simulink model "SpheroControl_CVT"  (R2014b)
settings: Solver=ode3  StartTime=0.0  StopTime=30  FixedStep=.2  RelTol=1e-3
InitFcn:
  | %sphName = uint8('Sphero-PGP');
  | 
  | move(char(sphName), 0, 0)
  | 
  | restartspeed = 65;
  | stopspeed = 1;
  | stopRadius = 50;
  | Kp = 0.2;
  |     Ki = 0;
  |     Kd = 0;
StopFcn:
  | %detectSpheroCVT( 10, 1);
  | 
  | move(sphName, 0, 0)
  | move(sphName, 0, 0, 0)
undefined symbols (not defined in the file or in its folder): IsPositionTracked, IsSkeletonTracked, JointDepthIndices, JointImageIndices, JointTrackingState, JointWorldCoordinates, none, PositionDepthIndices, PositionImageIndices, PositionWorldCoordinates, SegmentationData, SkeletonTrackingID, videoinput
libraries: visiontextngfix x1, imaqlib x1, aerolibanimutils x1, visionsinks x1
settings Model: Creator=dsethi  LastModifiedBy=dsethi
settings SolverCC: AlgebraicLoopSolver=LineSearch
settings DataIOCC: SignalLoggingSaveFormat=ModelDataLogs
settings DebuggingCC: MultiTaskDSMMsg=warning  MultiTaskCondExecSysMsg=none
settings RTWCC: IncludeERTFirstTime=on

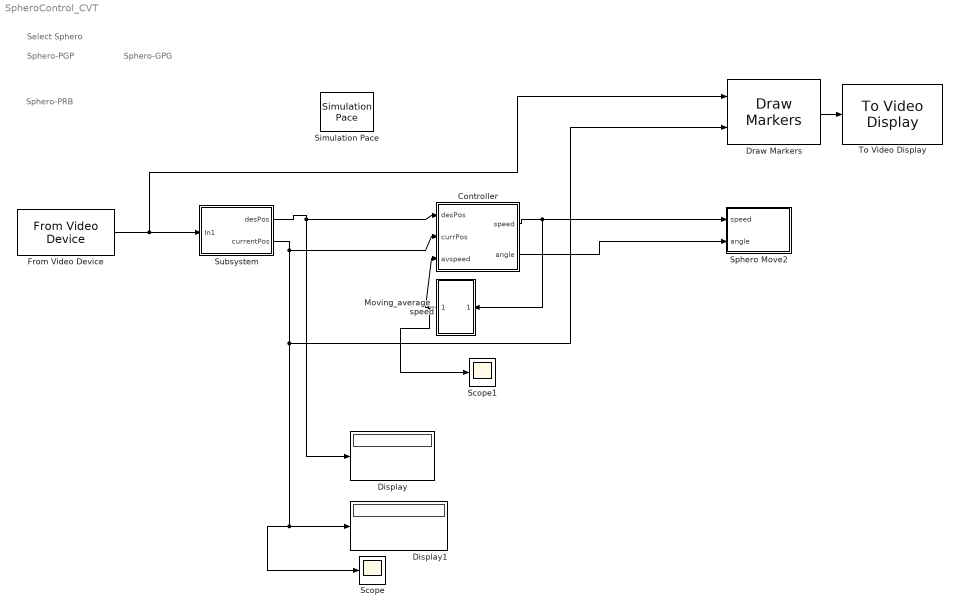
== system SpheroControl_CVT ==
  note: Select Sphero
  note: Sphero-PGP
  note: Sphero-GPG
  note: Sphero-PRB
  Controller : Stateflow chart  TreatAsAtomicUnit=on
  Display : Display
  Display1 : Display
  Draw Markers : visiontextngfix/Draw Markers  shape=X-mark  size=3  fill=off  fillClrSource=Specify via dialog  display=User-specified value  intensity=200  color=[255 0 0]  opacity=0.6  viewport=Entire image  antialiasing=off  inType=Obsolete  imagePorts=One multidimensional signal  prodOutputMode=Binary point scaling  prodOutputWordLength=32  prodOutputFracLength=14  memoryMode=Specify word length  memoryWordLength=16  memoryFracLength=15  roundingMode=Floor  overflowMode=off
  From Video Device : imaqlib/From Video Device  DeviceMenu=winvideo 1 (Microsoft LifeCam Cinema)  Device=winvideo 1 (Microsoft LifeCam Cinema)  ObjConstructor=videoinput('winvideo', 1)  VideoFormatMenu=MJPG_640x480  VideoFormat=MJPG_640x480  VideoSource=input1  ROIPosition=[0 0 480 640]  EnableHWTrigger=off  TriggerConfiguration=none/none  SampleTime=0.2  OutputPortsMode=One multidimensional signal  DataType=single  CanDoHWTrigger=no  ReturnedColorSpace=rgb  BlockHandle=1921.0006  ROIWidth=640  ROIHeight=480  ROIColumn=0  ROIRow=0  EngXMLPath=D:\jobarchive\R2014bd\2014_07_22_h06m43s29_job123_pass\matlab\toolbox\imaq\imaq\private  DevXMLPath=D:\jobarchive\R2014bd\2014_07_22_h06m43s29_job123_pass\matlab\toolbox\imaq\supportpackages\genericvideo\adaptor\win64  EngLibPath=D:\jobarchive\R2014bd\2014_07_22_h06m43s29_job123_pass\matlab\toolbox\imaq\imaqblks\imaqmex\win64  ColorSpace=rgb  BayerSensorAlignment=grbg  AllMetadata=IsPositionTracked;IsSkeletonTracked;JointDepthIndices;JointImageIndices;JointTrackingState;JointWorldCoordinates;PositionDepthIndices;PositionImageIndices;PositionWorldCoordinates;SegmentationData;SkeletonTrackingID
  Moving_average_speed : Subsystem
  Scope : Scope
      settings: SaveName=SpheroPos
  Scope1 : Scope
      settings: SaveName=movingAvg
  Simulation Pace : aerolibanimutils/Simulation Pace  SimulationPace=1  SleepMode=MATLAB Thread  OutputPaceError=off  SampleTime=-1
      settings: AttributesFormatString=%<SimulationPace> sec/sec
  Sphero Move2 : MATLAB Function  TreatAsAtomicUnit=on
  Subsystem : Subsystem  mask{cameraNum=Logitech, desPos=[200, 150]}
      mask prompts: cameraNum "Camera"; desPos "Desired position (x, y coordinates)"
      mask TypeOptions cameraNum: Logitech | Microsoft
  To Video Display : visionsinks/To Video Display  inputType=Obsolete  imagePorts=One multidimensional signal  OutputDevice=On-screen video monitor  fullScreen=off  videoWindowX=-7  videoWindowY=10  saveWindowSize=off  videoWindowWidth=640  videoWindowHeight=480  dataOrg=Column-major  openAtMdlStart=on  isWindowOpen=off  inputColorFormat=RGB
  wires:
  Subsystem/1(desPos) -> Display/1, Controller/1(desPos)
  Subsystem/2(currentPos) -> Controller/2(currPos), Scope/1, Display1/1, Draw Markers/2
  From Video Device/1 -> Draw Markers/1, Subsystem/1(In1)
  Draw Markers/1 -> To Video Display/1
  Controller/1(speed) -> Moving_average_speed/1(In1), Sphero Move2/1(speed)
  Controller/2(angle) -> Sphero Move2/2(angle)
  Moving_average_speed/1(Out1) -> Scope1/1, Controller/3(avspeed)

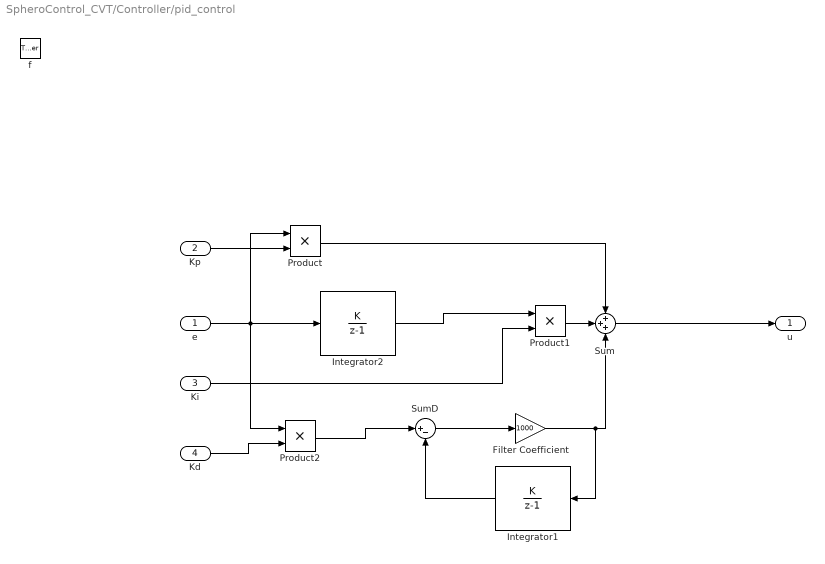
== system SpheroControl_CVT/Controller/pid_control ==
  e : Inport  OutDataTypeStr=double  PortDimensions=1
  Kp : Inport  Port=2  OutDataTypeStr=double  PortDimensions=1
  Ki : Inport  Port=3  OutDataTypeStr=double  PortDimensions=1
  Kd : Inport  Port=4  OutDataTypeStr=double  PortDimensions=1
  f : TriggerPort  TriggerType=function-call
      settings: CopyFcn=Stateflow.SLINSF.SimulinkMan.removeBlockPreDeleteFcn  PreDeleteFcn=Stateflow.SLINSF.SimulinkMan.unsafePredeleteFcn
  Filter Coefficient : Gain  Gain=1000
  Integrator1 : DiscreteIntegrator  IntegratorMethod=Accumulation: Forward Euler  InitialConditionSetting=State (most efficient)  SampleTime=-1
  Integrator2 : DiscreteIntegrator  IntegratorMethod=Accumulation: Forward Euler  InitialConditionSetting=State (most efficient)  SampleTime=-1
  Product : Product
  Product1 : Product
  Product2 : Product
  Sum : Sum  Inputs=+++
  SumD : Sum  DisableCoverage=on  Inputs=|+-
  u : Outport
  wires:
  Sum/1 -> u/1
  Product1/1 -> Sum/2
  Integrator1/1 -> SumD/2
  Filter Coefficient/1 -> Integrator1/1, Sum/3
  SumD/1 -> Filter Coefficient/1
  Product2/1 -> SumD/1
  Product/1 -> Sum/1
  e/1 -> Integrator2/1, Product2/1, Product/1
  Kp/1 -> Product/2
  Integrator2/1 -> Product1/1
  Ki/1 -> Product1/2
  Kd/1 -> Product2/2

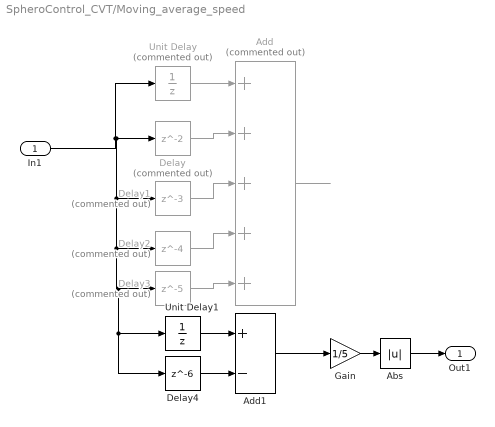
== system SpheroControl_CVT/Moving_average_speed ==
  In1 : Inport
  Abs : Abs
  Add : Sum  Commented=on  Inputs=+++++
  Add1 : Sum  Inputs=+-
  Delay : Delay  Commented=on
  Delay1 : Delay  Commented=on  DelayLength=3
  Delay2 : Delay  Commented=on  DelayLength=4
  Delay3 : Delay  Commented=on  DelayLength=5
  Delay4 : Delay  DelayLength=6
  Gain : Gain  Gain=1/5
  Unit Delay : UnitDelay  Commented=on  SampleTime=-1
  Unit Delay1 : UnitDelay  SampleTime=-1
  Out1 : Outport
  wires:
  Delay/1 -> Add/2
  In1/1 -> Unit Delay/1, Unit Delay1/1, Delay4/1, Delay3/1, Delay2/1, Delay1/1, Delay/1
  Unit Delay/1 -> Add/1
  Delay1/1 -> Add/3
  Delay2/1 -> Add/4
  Delay3/1 -> Add/5
  Add/1 -> ?
  Gain/1 -> Abs/1
  Delay4/1 -> Add1/2
  Add1/1 -> Gain/1
  Unit Delay1/1 -> Add1/1
  Abs/1 -> Out1/1

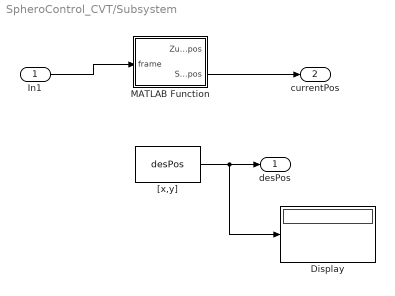
== system SpheroControl_CVT/Subsystem ==
  In1 : Inport
  Display : Display
  MATLAB Function : MATLAB Function  TreatAsAtomicUnit=on
  "[x,y]" : Constant  Value=desPos
  desPos : Outport
  currentPos : Outport  Port=2
  wires:
  "[x,y]"/1 -> Display/1, desPos/1
  In1/1 -> MATLAB Function/1(frame)
  MATLAB Function/2(Spheropos) -> currentPos/1

== matlab function SpheroControl_CVT/Subsystem/MATLAB Function ==
  data: frame input; Zumopos output single; Spheropos output
function [Zumopos, Spheropos] = fcn(frame)
%#codegen
persistent init

coder.extrinsic('detectMinions2')

Zumopos = single([0 0]);
Spheropos = [0; 0];

if isempty(init)
    [Zumopos, Spheropos] = detectMinions2(frame, 1);
    init = 1;
else
    [Zumopos, Spheropostemp] = detectMinions2(frame);
    Spheropos = Spheropostemp';
end

== stateflow chart SpheroControl_CVT/Controller ==
  state Control [parallel]
    settings: executionOrder=2
    state Motion
      en, du: speed = pid_control(dist, Kp, Ki, Kd);
    state Stop
      en, du: speed = 0;
    state Restart
      en, du: speed = restartspeed;
    (default) -> Motion
    Stop -> Motion [order 2] : [dist>stopRadius]
    Motion -> Stop [order 1] : [dist<stopRadius]
    Restart -> Motion [order 1] : [avspeed>stopspeed]
    Motion -> Restart [order 2] : [avspeed<stopspeed]
    Restart -> Stop [order 2] : [dist<stopRadius]
    Stop -> Restart [order 1] : [avspeed<stopspeed && dist>stopRadius]
  state ComputeDist [parallel]
    en, du: [dist, angle] = relativePos(desPos, currPos);
    settings: executionOrder=1
  state u = pid_control(e,Kp,Ki,Kd) [function]
  data: desiredPos function_input; currentPos function_input; distance function_output; angleOut function_output; e function_input double size=1; u function_output; Kp function_input double size=1; Ki function_input double size=1; Kd function_input double size=1; speed output; dist local; angle output; desPos input; currPos input; Kp parameter; Ki parameter; Kd parameter; avspeed input; stopspeed parameter; restartspeed parameter; stopRadius parameter
  function [distance, angleOut] = relativePos(desiredPos, currentPos):
    | function [distance, angleOut] = relativePos(desiredPos, currentPos)
    | 
    | coder.extrinsic('radtodeg', 'pdist')
    | distance = 0;
    | angleOut = 0;
    | 
    | if currPos(1)<0 || currPos(2)<0
    |     
    |     return
    | end
    | %% Angle and distance calculation
    |  
    |     %Angle of desired position wrt y axis (or orientation of sphero)
    |     angleOut = atan2(desiredPos(1)-currentPos(1), desiredPos(2)-currentPos(2));
    | 
    |     if angleOut<0
    |         angleOut = -angleOut;
    |     else
    |         angleOut = 2*pi-angleOut;
    |     end
    | 
    |     angleOut = radtodeg(angleOut);
    | 
    |     distance = pdist([desiredPos'; currentPos']); %Distance or the error

== matlab function SpheroControl_CVT/Sphero Move2 ==
  data: speed input; angle input; sphName parameter uint8
function fcn(speed, angle, sphName)
%#codegen
coder.extrinsic('move')

move(char(sphName), speed, angle);
